simulink model "testUSS"  (R2016a)
settings: Solver=FixedStepAuto  StartTime=0.0  StopTime=10.0  RelTol=1e-3
settings Model: SimulationMode=external  ExtModeTrigDuration=2  Creator=maste_000  LastModifiedBy=maste_000
settings OptimizationCC: OptimizeModelRefInitCode=on  LifeSpan=1  MaxStackSize=64
settings HardwareCC: ProdBitPerInt=16  ProdBitPerPointer=16  ProdLargestAtomicFloat=None  ProdWordSize=8  ProdHWDeviceType=Atmel->AVR
settings RTWCC: SystemTargetFile=ert.tlc  HardwareBoard=Arduino Mega 2560  TemplateMakefile=ert_default_tmf  GenerateReport=on  Toolchain=Arduino AVR v1.6.1  BuildConfiguration=Faster Runs  IncludeHyperlinkInReport=on  LaunchReport=on  GenerateTraceInfo=on  GenerateTraceReport=on  GenerateTraceReportSl=on  GenerateTraceReportSf=on  GenerateTraceReportEml=on
settings CodeAppCC: ForceParamTrailComments=on  IgnoreCustomStorageClasses=off  OperatorAnnotations=on  SimulinkDataObjDesc=on  SFDataObjDesc=on  MATLABFcnDesc=on  InsertBlockDesc=on  MATLABSourceComments=on
settings ERTTargetCC: SupportContinuousTime=on  SupportVariableSizeSignals=on

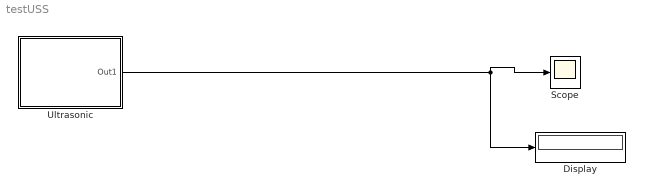
== system testUSS ==
  Display : Display
  Scope : Scope
  Ultrasonic : Subsystem  mask{useInch=off, pinNum=3, SampleTime=0.1}
      mask prompts: SampleTime "Simulink:blkprm_prompts:AllSrcBlksSampleTime"
      mask TypeOptions useInch: MATLAB System/useInch
      mask TypeOptions pinNum: MATLAB System/pinNum
      mask TypeOptions SampleTime: Constant/SampleTime
      mask Display: image('download (1).jpg');
  wires:
  Ultrasonic/1(Out1) -> Scope/1, Display/1

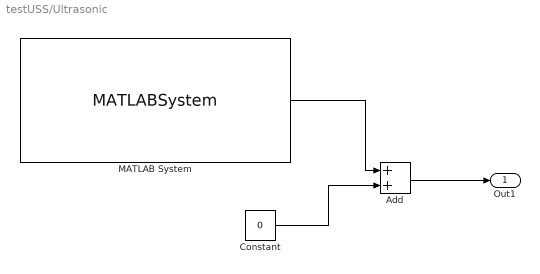
== system testUSS/Ultrasonic ==
  Add : Sum
  Constant : Constant  Value=0  SampleTime=SampleTime
  MATLAB System : MATLABSystem  System=arduino.USSensor  useInch=off  pinNum=pinNum  SimulateUsing=Interpreted execution
      mask Type: arduino.USSensor
      mask Display:
      | disp('USSensor');
      | port_label('output',1,'recordedDistance');
  Out1 : Outport
  wires:
  MATLAB System/1 -> Add/1
  Add/1 -> Out1/1
  Constant/1 -> Add/2
